simulink model "Discrete_System_1"  (R2023a)
settings: Solver=VariableStepAuto  StartTime=0.0  StopTime=10.0  RelTol=1e-3
settings Model: Creator=Aman  LastModifiedBy=Aman

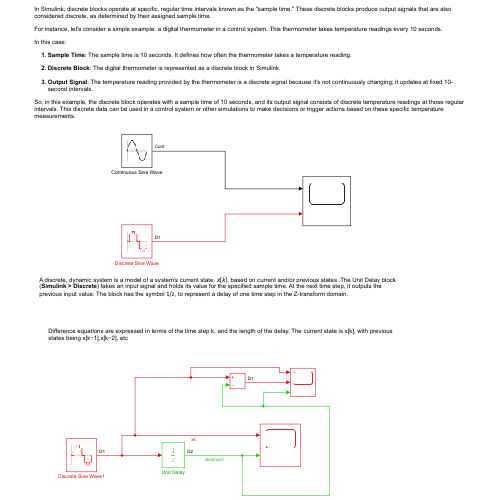
[thumbnail: Simulink's stored preview of the top-level diagram]
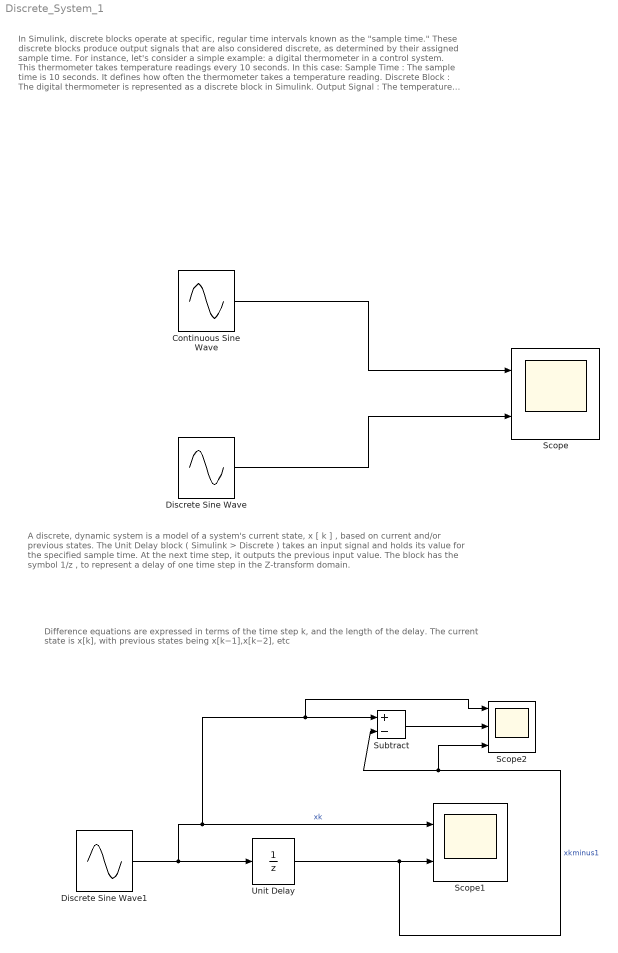
== system Discrete_System_1 ==
  note: Difference equations are expressed in terms of the time step k, and the length of the delay. The current state is x[k], with previous states being x[k−1],x[k−2], etc
  note: A discrete, dynamic system is a model of a system's current state, x [ k ] , based on current and/or previous states. The Unit Delay block ( Simulink > Discrete ) takes an input signal and holds its value for the specified sample time. At the next time step, it outputs the previous input value. The block has the symbol 1/z , to represent a delay of one time step in the Z-transform domain.
  note: In Simulink, discrete blocks operate at specific, regular time intervals known as the "sample time." These discrete blocks produce output signals that are also considered discrete, as determined by their assigned sample time.
      | For instance, let's consider a simple example: a digital thermometer in a control system. This thermometer takes temperature readings every 10 seconds.
      | In this case:
      | Sample Time : The sample time is 10 seconds. It defines how often the thermometer takes a temperature reading.
      | Discrete Block : The digital thermometer is represented as a discrete block in Simulink.
      | Output Signal : The temperature reading provided by the thermometer is a discrete signal because it's not continuously changing; it updates at fixed 10-second intervals.
      | So, in this example, the discrete block operates with a sample time of 10 seconds, and its output signal consists of discrete temperature readings at those regular intervals. This discrete data can be used in a control system or other simulations to make decisions or trigger actions based on these specific temperature measurements.
  Continuous Sine Wave : Sin  SampleTime=0
  Discrete Sine Wave : Sin  SampleTime=0.25
  Discrete Sine Wave1 : Sin  SampleTime=0.25
  Scope : Scope  NumInputPorts=2
  Scope1 : Scope  NumInputPorts=2
  Scope2 : Scope  NumInputPorts=3
  Subtract : Sum  Inputs=+-
  Unit Delay : UnitDelay  SampleTime=0.5  HasFrameUpgradeWarning=on
  wires:
  Continuous Sine Wave/1 -> Scope/1
  Discrete Sine Wave/1 -> Scope/2
  Discrete Sine Wave1/1 -> Subtract/1, Scope2/1, Scope1/1, Unit Delay/1  "xk"
  Unit Delay/1 -> Scope1/2, Scope2/3, Subtract/2  "xkminus1"
  Subtract/1 -> Scope2/2
